simulink model "six_phase_pmsm"  (Simulink 7.3)
settings: Solver=ode45  StartTime=0.0  StopTime=4  RelTol=1e-3
InitFcn:
  | % Processor selection for I/O assignment
  | % The chosen Target in the Coder Options window must match the selected MCU.
  | % Set the variable 'type_evm' to the following strings to choose a specific target:
  | 
  |   type_evm = 'TI28069';    % TI28069 Piccolo Launchpad
  | % type_evm = 'TI28377S';   % TI28377S Delfino Launchpad
  | % type_evm = 'TI28379LP';  % TI28379D Delfino Launchpad
  | % type_evm = 'TI280049C';  % TI280049C Piccolo Launchpad
  | % type_evm = 'TI28379CC';  % TI28379D Delfino Controlcard
  | % type_evm = 'TI28388D';   % TI28388D Controlcard
  | 
  | % -- IMPORTANT --
  | % For TI280049 Launchpad, make sure on the Launchpad switches S6, S8, S4 are set as 1, i.e. pushed to the dot side.
  | % And switch S3.1 also set as 1, i.e. pushed to BP (bypass) side.
  | 
  | 
  | % Configure I/O based on processor
  | switch (type_evm)
  | 	case 'TI28069'
  | 	% Configuration for TI28069 Launchpad
  | 	% On the Plant side
  | 		AO_RTBox_Is1 = [0,1];
  | 		AO_RTBox_Is2 = [2,3];
  | 		AO_RTBox_Vdc = [4,5];
  | 		ENC_RTBox_A = 6;
  | 		ENC_RTBox_B = 7;
  | 		ENC_RTBox_I = 23;
  | 		PWMCAP_RTBox_sw1 = [0:5];
  | 		PWMCAP_RTBox_sw2 = [16:21];
  | 		DO_RTBox_Eno = 4;
  | 		DI_RTBox_Power = 22;
  | 		AO_Vmax = 3.3;
  | 		AO_Factor = 1;
  | 
  | 	% On the MCU side
  | 		ADC_DSP_ADC = [7,9,2,10,0,8];
  | 		eQEP_DSP_eQEP = 1;
  | 		QEP_DSP_QEP = [50,51,53];
  | 		PWM_DSP_PWM1 = [1,2,3];
  | 		PWM_DSP_PWM2 = [4,5,6];
  | 		DO_DSP_LED = 34;
  | 		DI_DSP_En = 13;
  | 		PWR_DSP_GPIO = 27;
  | 		SCI_DSP = [28, 29];
  | 		ADC_Vmax = 3.3;
  | 
  | 	case 'TI28377S'
  | 	% Configuration for TI28377S Launchpad
  | 	% On the Plant side
  | 		AO_RTBox_Is1 = [4,6];
  | 		AO_RTBox_Is2 = [9,12];
  | 		AO_RTBox_Vdc = [14,10];
  | 		ENC_RTBox_A = 4;
  | 		ENC_RTBox_B = 5;
  | 		ENC_RTBox_I = 22;
  | 		PWMCAP_RTBox_sw1 = [16,17,18,19,0,1];
  | 		PWMCAP_RTBox_sw2 = [2,3,4,5,20,21];
  | 		DO_RTBox_Eno = 6;
  | 		DI_RTBox_Power = 26;
  | 		AO_Vmax = 3.3;
  | 		AO_Factor = 1;
  | 
  | 	% On the MCU side
  | 		ADC_DSP_ADC = [0,1,2,3,4,5];
  | 		eQEP_DSP_eQEP = 1;
  | 		QEP_DSP_QEP = [20,21,99];
  | 		PWM_DSP_PWM1 = [2,6,7];
  | 		PWM_DSP_PWM2 = [8,9,10];
  | 		DO_DSP_LED = 90; % Random GPIO since LED D9-D10 on Launchpad are controlled by GPIO12-13, which are already used as ePWM7A-B.
  | 		DI_DSP_En = 72;
  | 		PWR_DSP_GPIO = 43;
  | 		SCI_DSP = [85, 84];
  | 		ADC_Vmax = 3.3;
  | 
  | 	case 'TI28379LP'
  | 	% Configuration for TI28379D Launchpad
  | 	% On the Plant side
  | 		AO_RTBox_Is1 = [7,15];
  | 		AO_RTBox_Is2 = [6,3];
  | 		AO_RTBox_Vdc = [14,11];
  | 		ENC_RTBox_A = 4;
  | 		ENC_RTBox_B = 24;
  | 		ENC_RTBox_I = 22;
  | 		PWMCAP_RTBox_sw1 = [0:5];
  | 		PWMCAP_RTBox_sw2 = [16:21];
  | 		DO_RTBox_Eno = 6;
  | 		DI_RTBox_Power = 22;
  | 		AO_Vmax = 3.3;
  | 		AO_Factor = 1;
  | 
  | 	% On the MCU side
  | 		ADC_DSP_ADC = [0,1,2,3,4,5];
  | 		eQEP_DSP_eQEP = 2;
  | 		QEP_DSP_QEP = [24,25,26];
  | 		PWM_DSP_PWM1 = [1,2,3];
  | 		PWM_DSP_PWM2 = [4,5,6];
  | 		DO_DSP_LED = 34;
  | 		DI_DSP_En = 124;
  | 		PWR_DSP_GPIO = 66;
  | 		SCI_DSP = [43, 42];
  | 		ADC_Vmax = 3.3;
  | 
  | 	case 'TI280049C'
  | 	% Configuration for TI280049C Launchpad
  | 	% On the Plant side
  | 		AO_RTBox_Is1 = [15,7];
  | 		AO_RTBox_Is2 = [14,0];
  | 		AO_RTBox_Vdc = [8,6];
  | 		ENC_RTBox_A = 16;
  | 		ENC_RTBox_B = 17;
  | 		ENC_RTBox_I = 3;
  | 		PWMCAP_RTBox_sw1 = [0:5];
  | 		PWMCAP_RTBox_sw2 = [16:21];
  | 		DO_RTBox_Eno = 4;
  | 		DI_RTBox_Power = 24;
  | 		AO_Vmax = 3.3;
  | 
  | 	% On the MCU side
  | % -- IMPORTANT --
  | % For TI280049 Launchpad, make sure on the Launchpad switches S6, S8, S4 are set as 1, i.e. pushed to the dot side.
  | % And switch S3.1 also set as 1, i.e. pushed to BP (bypass) side.
  | 		ADC_DSP_ADC = [0,1,3,5,6,9];
  | 		eQEP_DSP_eQEP = 1;
  | 		QEP_DSP_QEP = [28,29,59];
  | 		PWM_DSP_PWM1 = [6,5,3];
  | 		PWM_DSP_PWM2 = [1,4,2];
  | 		DO_DSP_LED = 34;
  | 		DI_DSP_En = 58;
  | 		PWR_DSP_GPIO = 56;
  | 		SCI_DSP = [35, 37]; %Cannot use [28,29] since they are already used for eQEP1A-1B.
  | 		ADC_Vmax = 3.3;
  | 		AO_Factor = 1;
  | 
  | 	case 'TI28379CC'
  | 	% Configuration for TI28379D Controlcard
  | 	% On the Plant side
  |       AO_RTBox_Is1 = [15,13];
  | 		AO_RTBox_Is2 = [11,9];
  | 		AO_RTBox_Vdc = [7,5];
  | 		ENC_RTBox_A = 13;
  | 		ENC_RTBox_B = 14;
  | 		ENC_RTBox_I = 26;
  | 		PWMCAP_RTBox_sw1 = 0:5;
  | 		PWMCAP_RTBox_sw2 = 6:11;
  | 		DO_RTBox_Eno = 21;
  | 		DI_RTBox_Power = 14;
  | 		AO_Vmax = 5.0;
  | 		AO_Factor = 1.54; % breakout board scaling 6.8k/4.42k
  | 
  | 		% On the MCU side
  | 		ADC_DSP_ADC = 0:5;
  | 		eQEP_DSP_eQEP = 1;
  | 		QEP_DSP_QEP = [20,21,23];
  | 		PWM_DSP_PWM1 = [1,2,3];
  | 		PWM_DSP_PWM2 = [4,5,6];
  | 		DO_DSP_LED = 34;
  | 		DI_DSP_En = 40;
  | 		PWR_DSP_GPIO = 39;
  |       SCI_DSP = [28, 29];
  | 		ADC_Vmax = 3.0;
  | 
  | 
  | 	case 'TI28388D'
  | 	% Configuration for TI28388D Controlcard
  | 	% On the Plant side
  | 	   AO_RTBox_Is1 = [15,13];
  | 		AO_RTBox_Is2 = [11,9];
  | 		AO_RTBox_Vdc = [7,5];
  | 		ENC_RTBox_A = 13;
  | 		ENC_RTBox_B = 14;
  | 		ENC_RTBox_I = 26;
  | 		PWMCAP_RTBox_sw1 = 0:5;
  | 		PWMCAP_RTBox_sw2 = 6:11;
  | 		DO_RTBox_Eno = 21;
  | 		DI_RTBox_Power = 14;
  | 		AO_Vmax = 5.0;
  | 		AO_Factor = 1.54; % breakout board scaling 6.8k/4.42k
  | 
  | 		% On the MCU side
  | 		ADC_DSP_ADC = 0:5;
  | 		eQEP_DSP_eQEP = 1;
  | 		QEP_DSP_QEP = [20,21,23];
  | 		PWM_DSP_PWM1 = [1,2,3];
  | 		PWM_DSP_PWM2 = [4,5,6];
  | 		DO_DSP_LED = 34;
  | 		DI_DSP_En = 40;
  | 		PWR_DSP_GPIO = 39;
  |       SCI_DSP = [28, 29];
  | 		ADC_Vmax = 3.0;
  | 
  | 	otherwise
  | 	error('Unknown evaluation module selection, please choose either ''TI28069'', ''TI28377S'', ''TI28379LP'', ''TI280049C'', ''TI28379CC'' or ''TI28388D''.')
  | end
  | 
  | % Converter parameters
  | Vdc = 400; % DC source voltage in V
  | fsw = 10e3; % switching frequency in Hz
  | 
  | % Plant dicretizaton
  | Ts_plant = 7e-6; % sample step size of the plant subsystem in sec
  | 
  | % Controller dicretizaton
  | Ts_controller = 1/fsw; % sample step size of the control task in sec
  | 
  | % PMSM parameters
  | p = 3;
  | Zeta = pi/6;
  | Tsc=1e-4;
  | flux_magnet=0.7;
  | Ld=5e-3;
  | Lq=5e-3;
  | Lmd=3e-3;
  | Lmq=3e-3;
  | Ll = Ld-Lmd;
  | Rs=1.5;
  | J = 0.091*4;
  | 
  | % inverter d-q current control plant parameters
  | Rtot = Rs;
  | Lf_PI = Ld;
  | Rf_PI = Rtot;
  | K_plant = 1/Rf_PI;
  | T_plant = Lf_PI/Rf_PI;
  | Kpe = 1;
  | Tsw = 1/fsw;
  | Tpe = Tsw*1.5;
  | 
  | % d-q current controller PI design: Optimum Magnitude
  | Tn_PI = T_plant;
  | Ti_PI = 2*K_plant*Kpe*Tpe;
  | Kp_PI = Tn_PI/Ti_PI;
  | Ki_PI = 1/Ti_PI;
  | Kbc_PI = Ki_PI/Kp_PI;
  | 
  | kp_1d=Kp_PI;
  | ki_1d=Ki_PI;
  | kp_1q=Kp_PI;
  | ki_1q=Ki_PI;
  | kp_2d=Kp_PI;
  | ki_2d=Ki_PI;
  | kp_2q=Kp_PI;
  | ki_2q=Ki_PI;
  | 
  | 
  | %%
  | %%  ==> Enable the following commented section if there is a controls toolbox available with your installation of Matlab
  | %%
  | %% speed controller PI design: Symmetric optimum
  | %% Closed-loop current transfer function
  | %s = tf('s');
  | %Gcc = (Kp_PI+Ki_PI/s)*K_plant/(T_plant*s+1);
  | %w1 = 2*pi*10*fsw;
  | %[gain, ~] = bode(Gcc,w1);
  | %gaindB = 20*log10(gain);
  | %wg = 10^(log10(10*fsw*2*pi)+gaindB/20);
  | %Gi_fo = 1/(1/wg*s+1);  % First-order low-pass filter approximation of closed current control loop
  | % Controller design using bandwidth based crossover specifications
  | %wcw = 20; % Desired bandwidth of the speed control loop
  | %pm_w = 80*pi/180; % Desired phase-margin
  | %[magpw, phasepw] = bode(Gi_fo * 1/(s*J) * 3/2*p*flux_magnet,wcw);
  | %phasepw = phasepw*pi/180;
  | %Kp_w = -1/magpw*cos(pm_w-phasepw);
  | %Ti = 1/(-tan(pm_w-phasepw)*wcw);
  | %Ki_w = Kp_w/Ti;
  | %clear Gcc s Gi_fo
  | %%
  | %%   <== Comment end
  | %%
  | 
  | Kp_w =  2.2784
  | Ti =  0.29386
  | Ki_w =  7.7533
  | 
  | % Scaling
  | Vdc_scl = ADC_Vmax/2/Vdc;
  | Is_scl = ADC_Vmax/2/20;
  | Is_ofs = ADC_Vmax/2;
undefined symbols (not defined in the file): plecs
settings Model: Creator=kris  LastModifiedBy=manaswini  ExtModeTrigMode=oneshot  ExtModeArmWhenConnect=off  ExtModeAutoUpdateStatusClock=off
settings DataIOCC: LimitDataPoints=off  ReturnWorkspaceOutputs=off  SignalLoggingName=sigsOut
settings OptimizationCC: BooleanDataType=off  ExpressionDepthLimit=128  InitFltsAndDblsToZero=on
settings DebuggingCC: SaveWithParameterizedLinksMsg=none  SignalResolutionControl=TryResolveAllWithWarning  SolverPrmCheckMsg=none  MultiTaskDSMMsg=warning  MultiTaskCondExecSysMsg=none  FcnCallInpInsideContextMsg=Enable All  StrictBusMsg=ErrorLevel1
settings HardwareCC: TargetHWDeviceType=32-bit Generic  TargetUnknown=on  ProdEqTarget=off
settings RTWCC: IncludeERTFirstTime=on
settings CodeAppCC: CustomSymbolStrType=$N$R$M_T
settings GRTTargetCC: TargetFcnLib=ansi_tfl_tmw.mat  TargetFunctionLibrary=C89/C90 (ANSI)  ModelReferenceCompliant=off

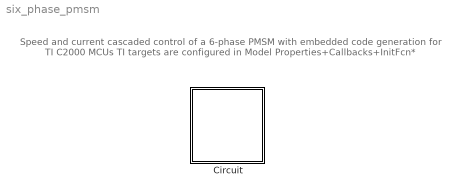
== system six_phase_pmsm ==
  note: Speed and current cascaded control of a 6-phase PMSM
      | with embedded code generation for TI C2000 MCUs
      | TI targets are configured in Model Properties+Callbacks+InitFcn*
  Circuit : Subsystem  LoadFcn=plecs('sl', 200);  InitFcn=plecs('sl', 214);  StartFcn=plecs('sl', 208);  StopFcn=plecs('sl', 209);  ClipboardFcn=plecs('sl', 212, 32);  mask(PlecsCircuit){PLECSData=<binary blob, 50192 chars, not shown>}
      mask prompts: PLECSData "PLECS Data (Do not delete or modify!)"
      mask help: Drag this block into a Simulink model to create a new electrical circuit.
      mask init:
      | % PLACE CUSTOM INITIALIZATIONS ABOVE
      | % DO NOT REMOVE
      | plecs('sl', 215);
      | % DO NOT REMOVE
      settings: CopyFcn=plecs('sl', 203);  DeleteFcn=plecs('sl', 205);  UndoDeleteFcn=plecs('sl', 206);  PreSaveFcn=plecs('sl', 211);  PostSaveFcn=plecs('sl', 201);  NameChangeFcn=plecs('sl', 210);  DestroyFcn=plecs('sl', 207);  PreCopyFcn=plecs('sl', 216);  OpenFcn=plecs('sl', 202);  ErrorFcn=plerrorfcn
      mask Display: disp('PLECS\nCircuit')

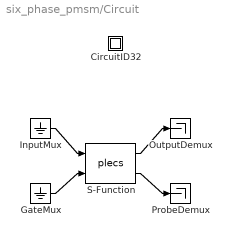
== system six_phase_pmsm/Circuit ==
  " CircuitID32 " : Subsystem
  " GateMux " : Ground
  " InputMux " : Ground
  " OutputDemux " : Terminator
  " ProbeDemux " : Terminator
  " S-Function " : S-Function  FunctionName=plecs  EnableBusSupport=off
  wires:
  " InputMux "/1 -> " S-Function "/1
  " GateMux "/1 -> " S-Function "/2
  " S-Function "/1 -> " OutputDemux "/1
  " S-Function "/2 -> " ProbeDemux "/1

== system six_phase_pmsm/Circuit/ CircuitID32  ==
